simulink model "SIRsimulink"  (R2018b)
settings: Solver=VariableStepAuto  StartTime=0.0  StopTime=300  RelTol=1e-3
values from neighbouring files (symbols this model uses):
  a = 1/9    (= 0.111111111111)    [SIR.m]    (also in prova esame.m = 0; soluzioni_2.m = -1; stabilita.m = 3)
  b = 0.35    [SIR.m]    (also in exe_vari_regressioe_autoval.m = A*ones(10,1); prova esame.m = [1 2 3]'; soluzioni_2.m = 1; soluzioni_3.m = sum(A,2))
  I = 1    [SIR.m]    (also in exe_vari_regressioe_autoval.m = eye(20))
  N = 7.8e9    (= 7800000000)    [SIR.m]
  R = 0    [SIR.m]    (also in exe_vari_regressioe_autoval.m = chol(A_1); prova esame.m = chol(B); rlc.m; soluzioni_3.m = chol(A))
  S = N - 1    (= 7799999999)    [SIR.m]    (also in stabilita.m = ss(A,B,C,D))
settings Model: Creator=Antonella  LastModifiedBy=Antonella

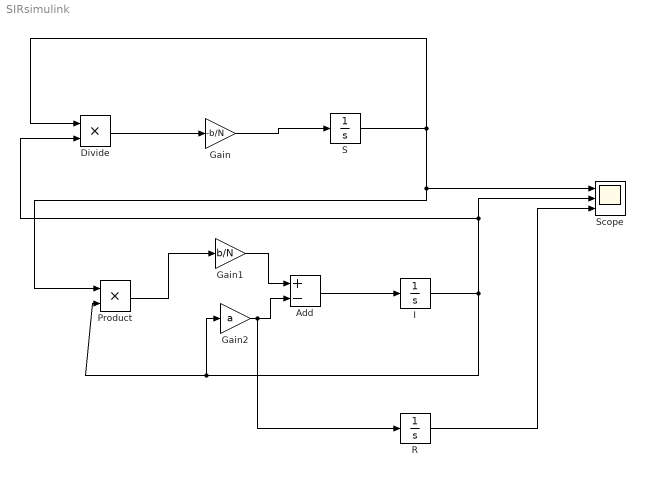
== system SIRsimulink ==
  Add : Sum  Inputs=+-
  Divide : Product  Inputs=**
  Gain : Gain  Gain=-b/N
  Gain1 : Gain  Gain=b/N
  Gain2 : Gain  Gain=a
  I : Integrator  InitialCondition=I
  Product : Product
  R : Integrator  InitialCondition=R
  S : Integrator  InitialCondition=S
  Scope : Scope  NumInputPorts=3
  wires:
  Gain/1 -> S/1
  Divide/1 -> Gain/1
  S/1 -> Product/1, Scope/1, Divide/1
  Product/1 -> Gain1/1
  I/1 -> Scope/2, Divide/2, Gain2/1, Product/2
  Gain1/1 -> Add/1
  Gain2/1 -> R/1, Add/2
  Add/1 -> I/1
  R/1 -> Scope/3
